simulink model "mck2_answer"  (R2019a)
settings: Solver=VariableStepAuto  StartTime=0.0  StopTime=10.0  RelTol=1e-3
PreLoadFcn:
  | m=0.1;
  | c=0.2;
  | k=0.5;
  | F=10;
settings Model: Creator=seong  LastModifiedBy=seong
settings DataIOCC: SaveFormat=Array  OutputSaveName=xout

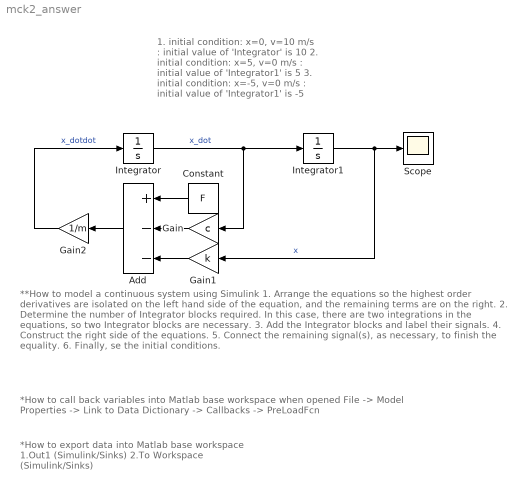
== system mck2_answer ==
  note: **How to model a continuous system using Simulink
      | 1. Arrange the equations so the highest order derivatives are isolated on the left hand side of the equation, and the remaining terms are on the right.
      | 2. Determine the number of Integrator blocks required. In this case, there are two integrations in the equations, so two Integrator blocks are necessary.
      | 3. Add the Integrator blocks and label their signals.
      | 4. Construct the right side of the equations.
      | 5. Connect the remaining signal(s), as necessary, to finish the equality.
      | 6. Finally, se the initial conditions.
  note: 1. initial condition: x=0, v=10 m/s
      | : initial value of 'Integrator' is 10
      | 2. initial condition: x=5, v=0 m/s
      | : initial value of 'Integrator1' is 5
      | 3. initial condition: x=-5, v=0 m/s
      | : initial value of 'Integrator1' is -5
  note: *How to export data into Matlab base workspace
      | 1.Out1 (Simulink/Sinks)
      | 2.To Workspace (Simulink/Sinks)
  note: *How to call back variables into Matlab base workspace when opened
      | File -> Model Properties -> Link to Data Dictionary -> Callbacks -> PreLoadFcn
  Add : Sum  Inputs=+--
  Constant : Constant  Value=F
  Gain : Gain  Gain=c
  Gain1 : Gain  Gain=k
  Gain2 : Gain  Gain=1/m
  Integrator : Integrator  InitialCondition=10
  Integrator1 : Integrator
  Scope : Scope
  wires:
  Integrator/1 -> Gain/1, Integrator1/1  "x_dot"
  Gain2/1 -> Integrator/1  "x_dotdot"
  Integrator1/1 -> Scope/1, Gain1/1  "x"
  Gain/1 -> Add/2
  Gain1/1 -> Add/3
  Add/1 -> Gain2/1
  Constant/1 -> Add/1
